simulink model "Rocket_sim"  (R2022a)
settings: Solver=VariableStepAuto  StartTime=0.0  StopTime=10.0  RelTol=1e-3
libraries: shared3dof x1, aerolibatmos2 x1
settings Model: Creator=jk111  LastModifiedBy=mt024518
settings DebuggingCC: UnconnectedInputMsg=warning  UnconnectedOutputMsg=warning  UnconnectedLineMsg=warning
settings RTWCC: DLArmComputeVersion=19.05

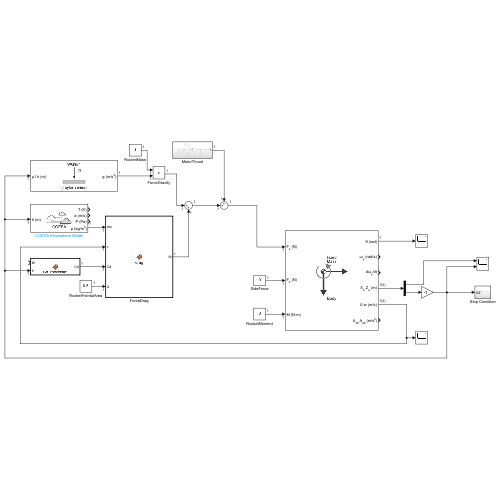
[thumbnail: Simulink's stored preview of the top-level diagram]
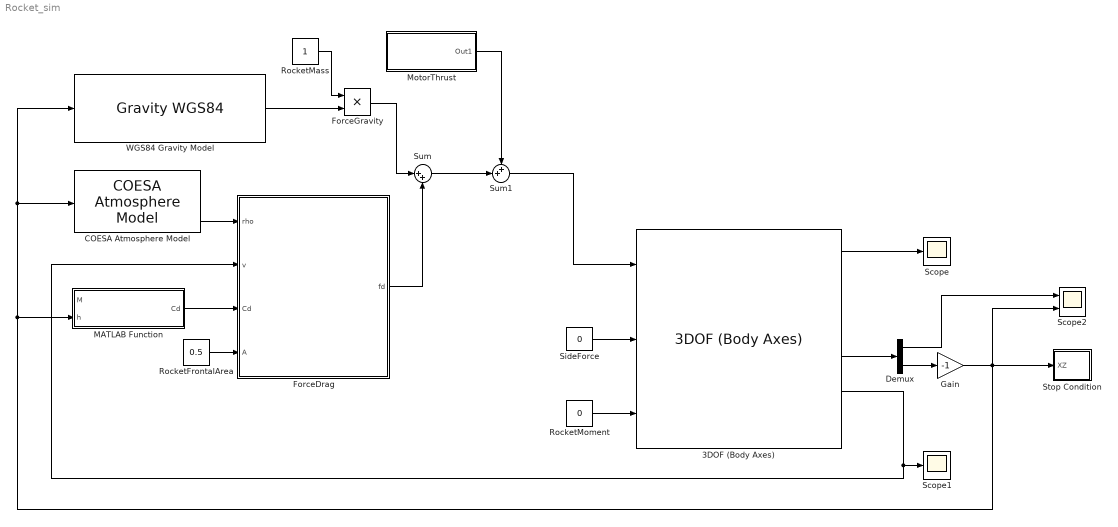
== system Rocket_sim ==
  3DOF (Body Axes) : shared3dof/3DOF (Body Axes)  units=Metric (MKS)  mtype=Fixed  v_ini=100  theta_ini=0  alpha_ini=0  pos_ini=[0 0]  q_ini=0  mass=1.0  mass_e=0.5  mass_f=3.0  Iyy=1.0  Iyy_e=0.5  Iyy_f=3.0  g_in=Internal  g=9.81  vre_flag=on  abi_flag=off  aMode=0  vel_statename=''  theta_statename=''  pos_statename=''  q_statename=''  mass_statename=''
      settings: SourceProductBaseCode=AE,PW,DR,MT,VE
  COESA Atmosphere Model : aerolibatmos2/COESA Atmosphere Model  units=Metric (MKS)  spec=1976 COESA-extended U.S. Standard Atmosphere  model=Profile  profile_var=High temperature  profile_percent=1%  profile_alt=5 km (16404 ft)  envelope_var=High temperature  envelope_percent=1%  action=Warning
  Demux : Demux  Outputs=2
  ForceDrag : MATLAB Function  TreatAsAtomicUnit=on
  ForceGravity : Product
  Gain : Gain  Gain=-1
  MATLAB Function : MATLAB Function  TreatAsAtomicUnit=on
  MotorThrust : Subsystem
  RocketFrontalArea : Constant  Value=0.5
  RocketMass : Constant
  RocketMoment : Constant  Value=0
  Scope : Scope
  Scope1 : Scope
  Scope2 : Scope  NumInputPorts=2
  SideForce : Constant  Value=0
  Stop Condition : Subsystem
  Sum : Sum  Inputs=|++
  Sum1 : Sum  Inputs=++|
  "WGS84 Gravity Model  " : GravityWGS84
  wires:
  SideForce/1 -> 3DOF (Body Axes)/2
  RocketMoment/1 -> 3DOF (Body Axes)/3
  RocketFrontalArea/1 -> ForceDrag/4(A)
  COESA Atmosphere Model/4 -> ForceDrag/1(rho)
  RocketMass/1 -> ForceGravity/1
  "WGS84 Gravity Model  "/1 -> ForceGravity/2
  ForceGravity/1 -> Sum/1
  ForceDrag/1(fd) -> Sum/2
  Sum1/1 -> 3DOF (Body Axes)/1
  Sum/1 -> Sum1/2
  MotorThrust/1(Out1) -> Sum1/1
  MATLAB Function/1(Cd) -> ForceDrag/3(Cd)
  3DOF (Body Axes)/1 -> Scope/1
  3DOF (Body Axes)/5 -> ForceDrag/2(v), Scope1/1
  3DOF (Body Axes)/4 -> Demux/1
  Demux/1 -> Scope2/1
  Demux/2 -> Gain/1
  Gain/1 -> MATLAB Function/2(h), "WGS84 Gravity Model  "/1, COESA Atmosphere Model/1, Scope2/2, Stop Condition/1(XZ)

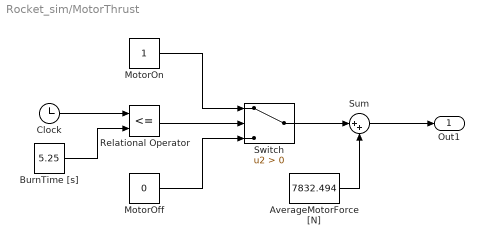
== system Rocket_sim/MotorThrust ==
  AverageMotorForce [N] : Constant  Value=7832.494
  BurnTime [s] : Constant  Value=5.25
  Clock : Clock
  MotorOff : Constant  Value=0
  MotorOn : Constant
  Relational Operator : RelationalOperator  Operator=<=  OutDataTypeStr=boolean  RndMeth=Simplest  InputSameDT=off
  Sum : Sum  Inputs=|++
  Switch : Switch  Criteria=u2 > Threshold  SaturateOnIntegerOverflow=off  InputSameDT=off
  Out1 : Outport
  wires:
  Switch/1 -> Sum/1
  Sum/1 -> Out1/1
  MotorOn/1 -> Switch/1
  MotorOff/1 -> Switch/3
  Relational Operator/1 -> Switch/2
  Clock/1 -> Relational Operator/1
  BurnTime [s]/1 -> Relational Operator/2
  AverageMotorForce [N]/1 -> Sum/2

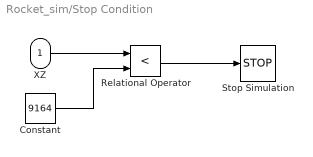
== system Rocket_sim/Stop Condition ==
  XZ : Inport
  Constant : Constant  Value=9164
  Relational Operator : RelationalOperator  Operator=<  OutDataTypeStr=boolean  RndMeth=Simplest  InputSameDT=off
  Stop Simulation : Stop
  wires:
  Relational Operator/1 -> Stop Simulation/1
  XZ/1 -> Relational Operator/1
  Constant/1 -> Relational Operator/2

== matlab function Rocket_sim/MATLAB Function ==
  data: M input; Cd output; h input
function Cd = Cd_rocketsim(M,h)

y = u;

== matlab function Rocket_sim/ForceDrag ==
  data: rho input; fd output; v input; Cd input; A input
function fd = drag(rho,v,Cd,A)

fd = (1/2)*rho*v^2*Cd*A;
